simulink library "IOlib"  (R2014a)
settings: Solver=ode45  SolverMode=SingleTasking  StartTime=0.0  StopTime=10.0  RelTol=1e-3
values from neighbouring files (symbols this model uses):
  tm = (tm_l + tm_r)./2    [AACplottingcode.m]    (also in AACplottingcode_Mzcurves.m = 0.0212; IMECE06plottingcode.m; If_alpha_tp_observer_shoreline.m)
  Ts = 0.002    [DSC_Control_Analysis.m]    (also in DSC_Control_Analysis_Exp.m; DSC_Speed_Control_Analysis.m; EC_params_nissan.m; Ext_MPCPara.m = SSD.Ts)
undefined symbols (not defined in the file or in its folder): Amps_per_volt, bs, Eff, eff, fs, gr, Js, Kf, Ki, kM, Kp, L, ljt, lma, lmt, lsa, R, rjt, rma, rmt, rsa
undefined symbols (not defined in the file): DataDescription
libraries: simulink x3, xpcdiamondlib x2, HardwareIO x2, NullHardware x1, PrerecordData x1, VehicleSimulation x1
(part 2 of 2)

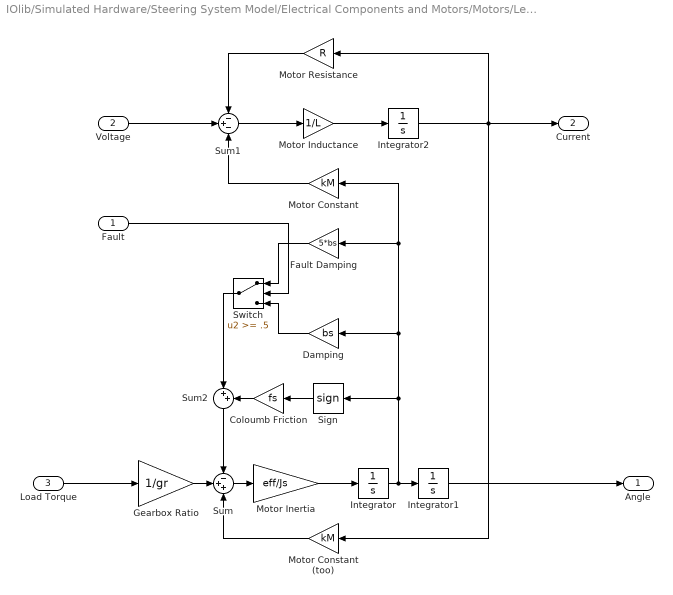
== system IOlib/Simulated Hardware/Steering System Model/Electrical Components and Motors/Motors/Left Motor ==
  Fault : Inport
  Voltage : Inport  Port=2
  Load Torque : Inport  Port=3
  Coloumb Friction : Gain  Gain=fs  SaturateOnIntegerOverflow=on  OutDataTypeStr=Inherit: Same as input  ParamDataTypeStr=Inherit: Same as input
  Damping : Gain  Gain=bs  SaturateOnIntegerOverflow=on  OutDataTypeStr=Inherit: Same as input  ParamDataTypeStr=Inherit: Same as input
  Fault Damping : Gain  Gain=5*bs  SaturateOnIntegerOverflow=on  OutDataTypeStr=Inherit: Same as input  ParamDataTypeStr=Inherit: Same as input
  Gearbox Ratio : Gain  Gain=1/gr  SaturateOnIntegerOverflow=on  OutDataTypeStr=Inherit: Same as input  ParamDataTypeStr=Inherit: Same as input
  Integrator : Integrator
  Integrator1 : Integrator  InitialCondition=.1*144*0
  Integrator2 : Integrator
  Motor Constant : Gain  Gain=kM  SaturateOnIntegerOverflow=on  OutDataTypeStr=Inherit: Same as input  ParamDataTypeStr=Inherit: Same as input
  Motor Constant (too) : Gain  Gain=kM  SaturateOnIntegerOverflow=on  OutDataTypeStr=Inherit: Same as input  ParamDataTypeStr=Inherit: Same as input
  Motor Inductance : Gain  Gain=1/L  SaturateOnIntegerOverflow=on  OutDataTypeStr=Inherit: Same as input  ParamDataTypeStr=Inherit: Same as input
  Motor Inertia : Gain  Gain=eff/Js  SaturateOnIntegerOverflow=on  OutDataTypeStr=Inherit: Same as input  ParamDataTypeStr=Inherit: Same as input
  Motor Resistance : Gain  Gain=R  SaturateOnIntegerOverflow=on  OutDataTypeStr=Inherit: Same as input  ParamDataTypeStr=Inherit: Same as input
  Sign : Signum  ZeroCross=off
  Sum : Sum  Inputs=-++  SaturateOnIntegerOverflow=on
  Sum1 : Sum  Inputs=-+-  SaturateOnIntegerOverflow=on
  Sum2 : Sum  Inputs=|++  SaturateOnIntegerOverflow=on
  Switch : Switch  Threshold=.5  ZeroCross=off  SaturateOnIntegerOverflow=on
  Angle : Outport
  Current : Outport  Port=2
  wires:
  Fault/1 -> Switch/2
  Fault Damping/1 -> Switch/1
  Damping/1 -> Switch/3
  Sum/1 -> Motor Inertia/1
  Motor Inertia/1 -> Integrator/1
  Integrator/1 -> Integrator1/1, Fault Damping/1, Motor Constant/1, Damping/1, Sign/1
  Integrator2/1 -> Current/1, Motor Constant (too)/1, Motor Resistance/1
  Motor Inductance/1 -> Integrator2/1
  Sum1/1 -> Motor Inductance/1
  Motor Resistance/1 -> Sum1/1
  Motor Constant/1 -> Sum1/3
  Voltage/1 -> Sum1/2
  Integrator1/1 -> Angle/1
  Gearbox Ratio/1 -> Sum/2
  Sign/1 -> Coloumb Friction/1
  Coloumb Friction/1 -> Sum2/2
  Sum2/1 -> Sum/1
  Switch/1 -> Sum2/1
  Motor Constant (too)/1 -> Sum/3
  Load Torque/1 -> Gearbox Ratio/1

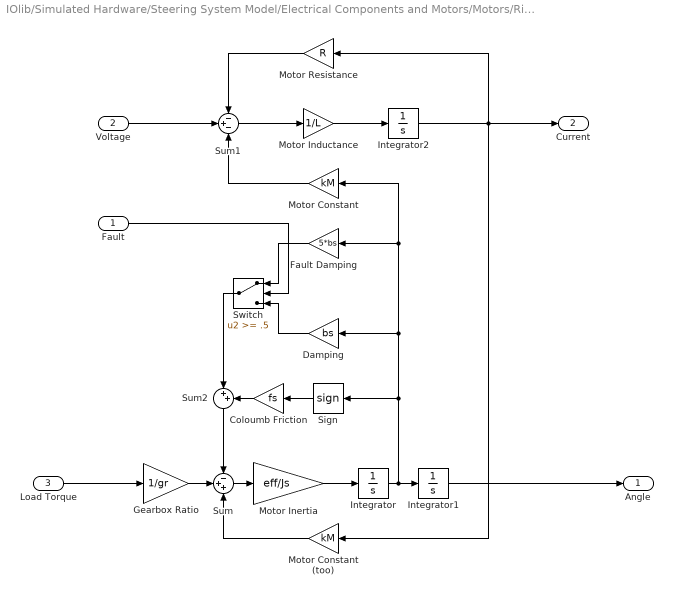
== system IOlib/Simulated Hardware/Steering System Model/Electrical Components and Motors/Motors/Right Motor ==
  Fault : Inport
  Voltage : Inport  Port=2
  Load Torque : Inport  Port=3
  Coloumb Friction : Gain  Gain=fs  SaturateOnIntegerOverflow=on  OutDataTypeStr=Inherit: Same as input  ParamDataTypeStr=Inherit: Same as input
  Damping : Gain  Gain=bs  SaturateOnIntegerOverflow=on  OutDataTypeStr=Inherit: Same as input  ParamDataTypeStr=Inherit: Same as input
  Fault Damping : Gain  Gain=5*bs  SaturateOnIntegerOverflow=on  OutDataTypeStr=Inherit: Same as input  ParamDataTypeStr=Inherit: Same as input
  Gearbox Ratio : Gain  Gain=1/gr  SaturateOnIntegerOverflow=on  OutDataTypeStr=Inherit: Same as input  ParamDataTypeStr=Inherit: Same as input
  Integrator : Integrator
  Integrator1 : Integrator  InitialCondition=0.1*144*0
  Integrator2 : Integrator
  Motor Constant : Gain  Gain=kM  SaturateOnIntegerOverflow=on  OutDataTypeStr=Inherit: Same as input  ParamDataTypeStr=Inherit: Same as input
  Motor Constant (too) : Gain  Gain=kM  SaturateOnIntegerOverflow=on  OutDataTypeStr=Inherit: Same as input  ParamDataTypeStr=Inherit: Same as input
  Motor Inductance : Gain  Gain=1/L  SaturateOnIntegerOverflow=on  OutDataTypeStr=Inherit: Same as input  ParamDataTypeStr=Inherit: Same as input
  Motor Inertia : Gain  Gain=eff/Js  SaturateOnIntegerOverflow=on  OutDataTypeStr=Inherit: Same as input  ParamDataTypeStr=Inherit: Same as input
  Motor Resistance : Gain  Gain=R  SaturateOnIntegerOverflow=on  OutDataTypeStr=Inherit: Same as input  ParamDataTypeStr=Inherit: Same as input
  Sign : Signum  ZeroCross=off
  Sum : Sum  Inputs=-++  SaturateOnIntegerOverflow=on
  Sum1 : Sum  Inputs=-+-  SaturateOnIntegerOverflow=on
  Sum2 : Sum  Inputs=|++  SaturateOnIntegerOverflow=on
  Switch : Switch  Threshold=.5  ZeroCross=off  SaturateOnIntegerOverflow=on
  Angle : Outport
  Current : Outport  Port=2
  wires:
  Load Torque/1 -> Gearbox Ratio/1
  Motor Constant (too)/1 -> Sum/3
  Switch/1 -> Sum2/1
  Sum2/1 -> Sum/1
  Coloumb Friction/1 -> Sum2/2
  Sign/1 -> Coloumb Friction/1
  Gearbox Ratio/1 -> Sum/2
  Integrator1/1 -> Angle/1
  Voltage/1 -> Sum1/2
  Motor Constant/1 -> Sum1/3
  Motor Resistance/1 -> Sum1/1
  Sum1/1 -> Motor Inductance/1
  Motor Inductance/1 -> Integrator2/1
  Integrator2/1 -> Motor Resistance/1, Motor Constant (too)/1, Current/1
  Integrator/1 -> Sign/1, Damping/1, Motor Constant/1, Fault Damping/1, Integrator1/1
  Motor Inertia/1 -> Integrator/1
  Sum/1 -> Motor Inertia/1
  Damping/1 -> Switch/3
  Fault Damping/1 -> Switch/1
  Fault/1 -> Switch/2
